simulink model "solarboat_1d_sim"  (R2022a)
settings: Solver=FixedStepAuto  StartTime=0.0  StopTime=5.0  FixedStep=0.00001  RelTol=1e-3
values from neighbouring files (symbols this model uses):
  Dp = 0.4    [params.mat]
  rho = 1020    [params.mat]
libraries: fl_lib x7, nesl_utility x5, ee_lib x2
settings Model: Creator=Shotaro Itahara  LastModifiedBy=Shotaro Itahara

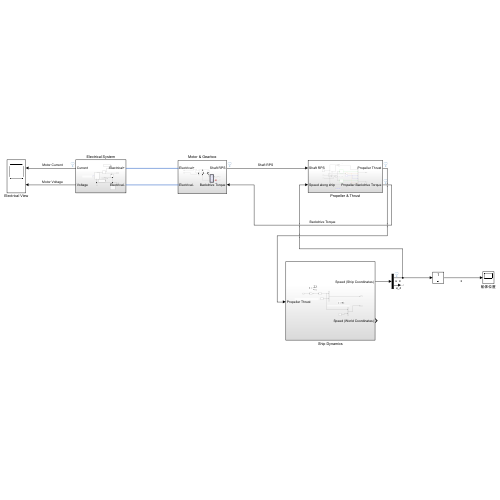
[thumbnail: Simulink's stored preview of the top-level diagram]
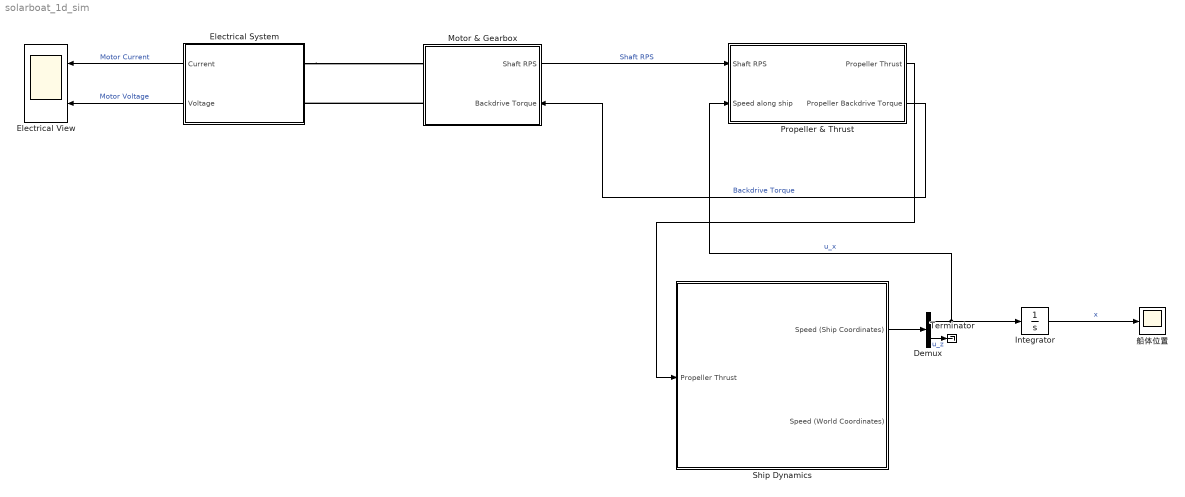
== system solarboat_1d_sim ==
  Demux : Demux  Outputs=2
  Electrical System : Subsystem
  Electrical View : Scope  NumInputPorts=2
  Integrator : Integrator
  Motor & Gearbox : Subsystem
      settings: PortSchema="{\"entries\":[{\"content\":{\"sides\":[{\"content\":{\"connectorIds\":[\"LConn1\",\"LConn2\"]},\"type\":\"ConnectorPlacement.EquallySpacedRectSide\",\"uuid\":\"90ac90da-f4b1-4979-b766-f3e8a99432da\"},{\"content\":{\"connectorIds\":[\"Out1\",\"In1\"],\"side\":\"RIGHT\"},\"type\":\"ConnectorPlacement.EquallySpacedRectSide\",\"uuid\":\"f54fcc4a-87d0-402f-8928-be8d6399a7de\"},{\"content\":{\"connectorIds\":[],\"side\":\"TOP\"},\"type\":\"ConnectorPlacement.EquallySpacedRectSide\",\"uuid\":\"30ecd799-1637-4d93-8d9a-4e0fe730cc63\"},{\"content\":{\"connectorIds\":[],\"side\":\"BOTTOM\"},\"type\":\"ConnectorPlacement.EquallySpacedRectSide\",\"uuid\":\"8dd49e10-c2e0-4b3a-8c8a-c1b45edb990f\"}]},\"type\":\"ConnectorPlacement.EquallySpacedConnector\",\"uuid\":\"f75a9819-a321-498b-8a3b-fea3fe879552\"}],\"packageUris\":[\"http://schema.mathworks.com/mf0/Connector/R2020b\"],\"version\":\"1.0\"}"
  Propeller & Thrust : Subsystem
  Ship Dynamics : Subsystem
  Terminator : Terminator
  船体位置 : Scope
  wires:
  Electrical System/1(Current) -> Electrical View/1  "Motor Current"
  Electrical System/2(Voltage) -> Electrical View/2  "Motor Voltage"
  Motor & Gearbox/1(Shaft RPS) -> Propeller & Thrust/1(Shaft RPS)  "Shaft RPS"
  Propeller & Thrust/2(Propeller Backdrive Torque) -> Motor & Gearbox/1(Backdrive Torque)  "Backdrive Torque"
  Ship Dynamics/1(Speed (Ship Coordinates)) -> Demux/1
  Demux/1 -> Integrator/1, Propeller & Thrust/2(Speed along ship)  "u_x"
  Propeller & Thrust/1(Propeller Thrust) -> Ship Dynamics/1(Propeller Thrust)
  Demux/2 -> Terminator/1  "u_z"
  Integrator/1 -> 船体位置/1  "x"
  connections:
  Electrical System/LConn1 -- Motor & Gearbox/LConn1
  Motor & Gearbox/LConn2 -- Electrical System/LConn2

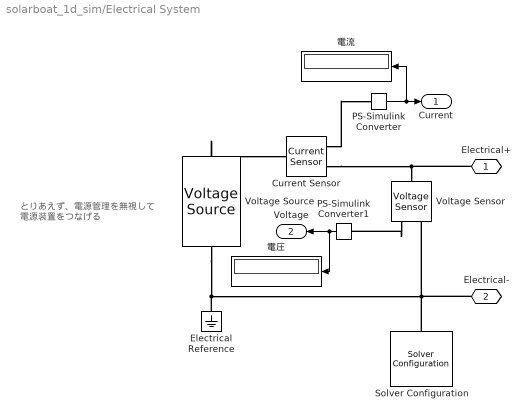
== system solarboat_1d_sim/Electrical System ==
  note: とりあえず、電源管理を無視して
      | 電源装置をつなげる
  Current Sensor : fl_lib/Electrical/Electrical Sensors/Current Sensor
      settings: SourceProductBaseCode=PW,SS,VE
  Electrical Reference : fl_lib/Electrical/Electrical Elements/Electrical Reference
      settings: SourceProductBaseCode=PW,SS,VE
  PS-Simulink Converter : nesl_utility/PS-Simulink Converter  PhysicalDomain=network_engine_domain  SubClassName=ps_output  LeftPortType=input  RightPortType=output  PseudoPeriodic=off  Frequencies=[]  VectorFormat=inherit  Unit=inherit  AffineConversion=off
      settings: SourceProductBaseCode=SS,PW,VE
  PS-Simulink Converter1 : nesl_utility/PS-Simulink Converter  PhysicalDomain=network_engine_domain  SubClassName=ps_output  LeftPortType=input  RightPortType=output  PseudoPeriodic=off  Frequencies=[]  VectorFormat=inherit  Unit=V  AffineConversion=off
      settings: SourceProductBaseCode=SS,PW,VE
  Solver Configuration : nesl_utility/Solver Configuration  PhysicalDomain=network_engine_domain  SubClassName=solver  LeftPortType=input  RightPortType=generic  Tones=[]  Harmonics=[]  SimulateNoise=off  Profile=off  UseLocalSampling=off  EnableSwitchedLinearOptims=on  FrequencyDomain=off  UseCCode=off  RelTol=0.001  AbsTol=0.001  MinStep=1e-09  ToWorkspace=off  RevertToSquareIcSolve=off  NumHomotopyIterations=100  PhasorMode=off  PhasorModeNumHarmonics=1  IndexReductionMethod=DerivativeReplacement  DoDC=off  ResidualTolerance=1e-09  UseLocalSolver=off  LocalSolverChoice=NE_BACKWARD_EULER_ADVANCER  LocalSolverSampleTime=0.001  DoFixedCost=off  MaxNonlinIter=3  MaxModeIter=2  ComputeImpulses=off  ImpulseIterations=2  LinearAlgebra=auto  LinearAlgebraNumThread=0  EquationFormulation=NE_TIME_EF  DelaysMemoryBudget=1024  AutomaticFiltering=off  FilteringTimeConstant=0.001  PartitionStorageMethod=AS_NEEDED  PartitionMemoryBudget=1024  PartitionMethod=ROBUST
      settings: SourceProductBaseCode=SS,PW,VE
  Voltage Sensor : fl_lib/Electrical/Electrical Sensors/Voltage Sensor
      settings: SourceProductBaseCode=PW,SS,VE
  Voltage Source : ee_lib/Sources/Voltage Source  dc_voltage=48 V  ac_voltage=0 V  ac_shift=0 rad  ac_frequency=60 Hz  noise_mode=0  PSD=0 V^2/Hz  repeatability=1  auto_seed=3499211588  user_seed=0  sample_time=1e-3 s  i_specify=off  i_priority=None  i=0 A  i_nominal_specify=off  i_nominal_unit=A  i_nominal_value=1  v_specify=off  v_priority=None  v=0 V  v_nominal_specify=off  v_nominal_unit=V  v_nominal_value=1
  電圧 : Display
  電流 : Display
  Electrical+ : PMIOPort  Side=Left
  Electrical- : PMIOPort  Port=2  Side=Left
  Current : Outport
  Voltage : Outport  Port=2
  wires:
  PS-Simulink Converter/1 -> 電流/1, Current/1
  PS-Simulink Converter1/1 -> 電圧/1, Voltage/1
  connections:
  Current Sensor/RConn2 -- Electrical+/RConn1 -- Voltage Sensor/LConn1
  Voltage Source/RConn1 -- Electrical Reference/LConn1 -- Voltage Sensor/RConn2 -- Electrical-/RConn1 -- Solver Configuration/RConn1
  Voltage Source/LConn1 -- Current Sensor/LConn1
  Current Sensor/RConn1 -- PS-Simulink Converter/LConn1
  Voltage Sensor/RConn1 -- PS-Simulink Converter1/LConn1

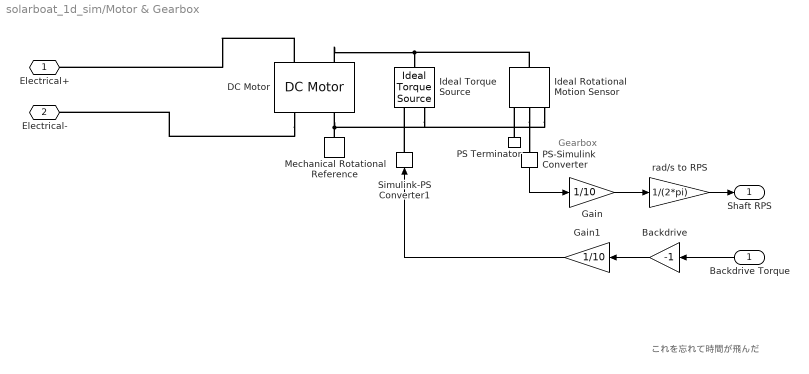
== system solarboat_1d_sim/Motor & Gearbox ==
  note: これを忘れて時間が飛んだ
  note: Gearbox
  Backdrive Torque : Inport
  Backdrive : Gain  Gain=-1
  DC Motor : ee_lib/Electromechanical/Brushed Motors/DC Motor  field_option=ee.enum.field_option.pm  Rf=100 Ohm  Lf=1 H  Laf=0.15 H  If0=0 A  parameterization=ee.enum.dcparam_option.load_speed  Ra=3.9 Ohm  La=1.2 H  emf_or_torque=ee.enum.emf_or_torque.kv  Kv=0.072e-3 V/rpm  Ki=6.876e-4 N*m/A  T_stall=0.24e-3 N*m  w_max=2880 rpm  w_rated=2879 rpm  P_rated=500 W  V_rated=24 V  lam_param=ee.enum.lam_param.damping  i_noload=0 A  V_i_noload=1.5 V  J=0.01 kg*m^2  lam=0 N*m*s/rad  speed0=1 rpm  enable_fault_armature=simscape.enum.onoff.off  rev_faulted=1 / 3  G_faulted_armature=1e-5 S  fault_trigger_armature=ee.enum.faults.faultTrigger.temporal  t_fault_armature=1 s  max_permissible_current_armature=inf A  t_fail_on_current_armature=1 s  enable_fault_field=simscape.enum.onoff.off  G_faulted_field=1e-5 S  fault_trigger_field=ee.enum.faults.faultTrigger.temporal  t_fault_field=1 s  max_permissible_current_field=inf A  t_fail_on_current_field=1 s  fault_action=simscape.enum.assert.action.none  alpha=3.93e-3 1/K  Tmeas=25 degC  thermal_mass=100 J/K  initial_temperature=25 degC
  Gain : Gain  Gain=1/10
  Gain1 : Gain  Gain=1/10
  Ideal Rotational Motion Sensor : fl_lib/Mechanical/Mechanical Sensors/Ideal Rotational Motion Sensor  wrap_angle=simscape.enum.onoff.off  offset=0 rad
      settings: SourceProductBaseCode=PW,SS,VE
  Ideal Torque Source : fl_lib/Mechanical/Mechanical Sources/Ideal Torque Source
      settings: SourceProductBaseCode=PW,SS,VE
  Mechanical Rotational Reference : fl_lib/Mechanical/Rotational Elements/Mechanical Rotational Reference
      settings: SourceProductBaseCode=PW,SS,VE
  PS Terminator : fl_lib/Physical Signals/Sinks/PS Terminator
      settings: SourceProductBaseCode=PW,SS,VE
  PS-Simulink Converter : nesl_utility/PS-Simulink Converter  PhysicalDomain=network_engine_domain  SubClassName=ps_output  LeftPortType=input  RightPortType=output  PseudoPeriodic=off  Frequencies=[]  VectorFormat=inherit  Unit=rad/s  AffineConversion=off
      settings: SourceProductBaseCode=SS,PW,VE
  Simulink-PS Converter1 : nesl_utility/Simulink-PS Converter  PhysicalDomain=network_engine_domain  SubClassName=ps_input  LeftPortType=input  RightPortType=output  PseudoPeriodic=off  Frequencies=[]  NoiseDistribution=none  NoiseParameters=[]  Unit=N*m  AffineConversion=off  FilteringAndDerivatives=provide  SimscapeFilterOrder=1  InputFilterTimeConstant=0.001  UdotUserProvided=0
      settings: SourceProductBaseCode=SS,PW,VE
  rad/s to RPS : Gain  Gain=1/(2*pi)
  Electrical+ : PMIOPort  Side=Left
  Electrical- : PMIOPort  Port=2  Side=Left
  Shaft RPS : Outport
  wires:
  PS-Simulink Converter/1 -> Gain/1
  Gain1/1 -> Simulink-PS Converter1/1
  Gain/1 -> rad/s to RPS/1
  Backdrive Torque/1 -> Backdrive/1
  rad/s to RPS/1 -> Shaft RPS/1
  Backdrive/1 -> Gain1/1
  connections:
  DC Motor/LConn2 -- Ideal Rotational Motion Sensor/LConn1 -- Ideal Torque Source/LConn1
  Mechanical Rotational Reference/LConn1 -- Ideal Rotational Motion Sensor/RConn1 -- Ideal Torque Source/RConn2 -- DC Motor/RConn2
  PS Terminator/LConn1 -- Ideal Rotational Motion Sensor/RConn3
  Ideal Rotational Motion Sensor/RConn2 -- PS-Simulink Converter/LConn1
  Simulink-PS Converter1/RConn1 -- Ideal Torque Source/RConn1
  DC Motor/RConn1 -- Electrical-/RConn1
  DC Motor/LConn1 -- Electrical+/RConn1

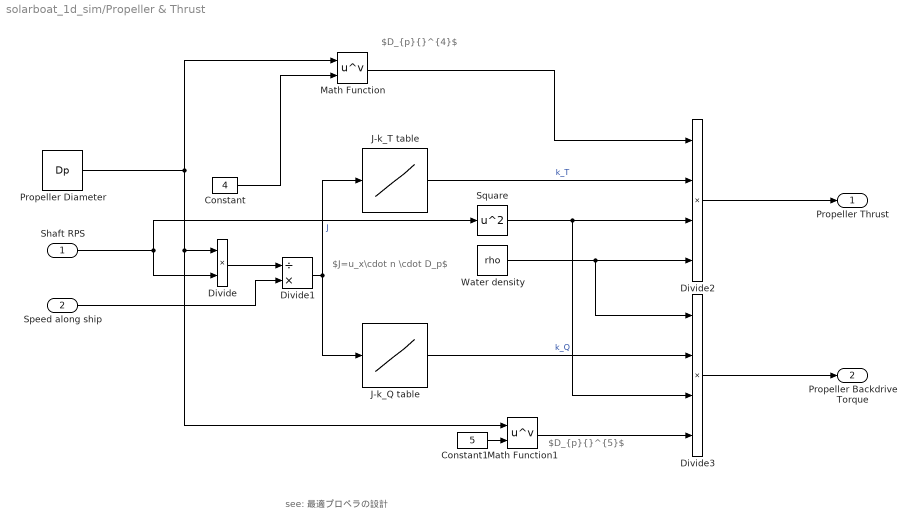
== system solarboat_1d_sim/Propeller & Thrust ==
  note: $J=u_x\cdot n \cdot D_p$
  note: $D_{p}{}^{4}$
  note: see: 最適プロペラの設計
  note: $D_{p}{}^{5}$
  Shaft RPS : Inport
  Speed along ship : Inport  Port=2
  Constant : Constant  Value=4
  Constant1 : Constant  Value=5
  Divide : Product  Inputs=**
  Divide1 : Product  Inputs=/*
  Divide2 : Product  Inputs=****
  Divide3 : Product  Inputs=****
  J-k_Q table : Lookup_n-D  NumberOfTableDimensions=1  BreakpointsForDimension1=[0.3,1]  Table=[0.06,0.01]  ExtrapMethod=Clip  UseLastTableValue=on  InternalRulePriority=Speed  RndMeth=Simplest
  J-k_T table : Lookup_n-D  NumberOfTableDimensions=1  BreakpointsForDimension1=[0.3;1]  Table=[0.4;0]  ExtrapMethod=Clip  UseLastTableValue=on  InternalRulePriority=Speed  RndMeth=Simplest
  Math Function : Math  Operator=pow
  Math Function1 : Math  Operator=pow
  Propeller Diameter : Constant  Value=Dp
  Square : Math  Operator=square
  Water density : Constant  Value=rho
  Propeller Thrust : Outport
  Propeller Backdrive Torque : Outport  Port=2
  wires:
  Propeller Diameter/1 -> Math Function1/1, Divide/1, Math Function/1
  Shaft RPS/1 -> Divide/2, Square/1
  Divide/1 -> Divide1/1
  Speed along ship/1 -> Divide1/2
  Divide1/1 -> J-k_Q table/1, J-k_T table/1  "J"
  J-k_T table/1 -> Divide2/2  "k_T"
  J-k_Q table/1 -> Divide3/2  "k_Q"
  Constant/1 -> Math Function/2
  Square/1 -> Divide3/3, Divide2/3
  Math Function/1 -> Divide2/1
  Divide2/1 -> Propeller Thrust/1
  Water density/1 -> Divide3/1, Divide2/4
  Constant1/1 -> Math Function1/2
  Math Function1/1 -> Divide3/4
  Divide3/1 -> Propeller Backdrive Torque/1

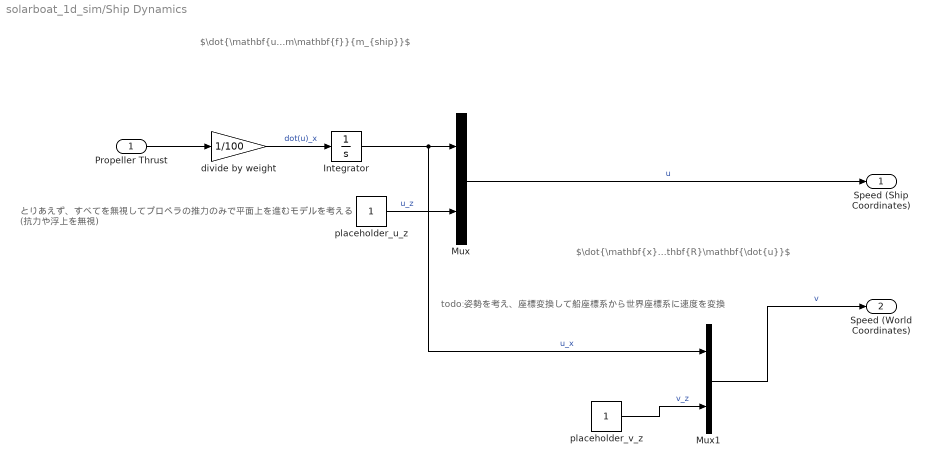
== system solarboat_1d_sim/Ship Dynamics ==
  note: とりあえず、すべてを無視してプロペラの推力のみで平面上を進むモデルを考える
      | (抗力や浮上を無視)
  note: todo:姿勢を考え、座標変換して船座標系から世界座標系に速度を変換
  note: $\dot{\mathbf{x}}=\mathbf{R}\mathbf{\dot{u}}$
  note: $\dot{\mathbf{u}}=\frac{\sum\mathbf{f}}{m_{ship}}$
  Propeller Thrust : Inport
  Integrator : Integrator
  Mux : Mux  Inputs=2
  Mux1 : Mux  Inputs=2
  divide by weight : Gain  Gain=1/100
  placeholder_u_z : Constant
  placeholder_v_z : Constant
  Speed (Ship Coordinates) : Outport
  Speed (World Coordinates) : Outport  Port=2
  wires:
  divide by weight/1 -> Integrator/1  "dot(u)_x"
  placeholder_u_z/1 -> Mux/2  "u_z"
  Mux/1 -> Speed (Ship Coordinates)/1  "u"
  placeholder_v_z/1 -> Mux1/2  "v_z"
  Mux1/1 -> Speed (World Coordinates)/1  "v"
  Propeller Thrust/1 -> divide by weight/1
  Integrator/1 -> Mux1/1, Mux/1  "u_x"
